simulink model "pendule_inv_capteur_etu"  (R2021a)
settings: Solver=VariableStepAuto  StartTime=0.0  StopTime=100  RelTol=1e-3
values from neighbouring files (symbols this model uses):
  K = [10 1]    [simu_pendule_inv_capteur_etu.m]    (also in simu_pendule_inv_echant_etu.m = [30 10]; simu_pendule_inv_etu.m = [30 10])
  ue = 0    [simu_pendule_inv_capteur_etu.m]    (also in simu_pendule_inv_echant_etu.m; simu_pendule_inv_etu.m)
  x0 = [pi/20 0]'    [simu_pendule_inv_capteur_etu.m]    (also in simu_pendule_inv_echant_etu.m; simu_pendule_inv_etu.m = [pi/10 0]')
  xe = [0 0]'    [simu_pendule_inv_capteur_etu.m]    (also in simu_pendule_inv_echant_etu.m; simu_pendule_inv_etu.m)
settings Model: Creator=ialouane  LastModifiedBy=ialouane

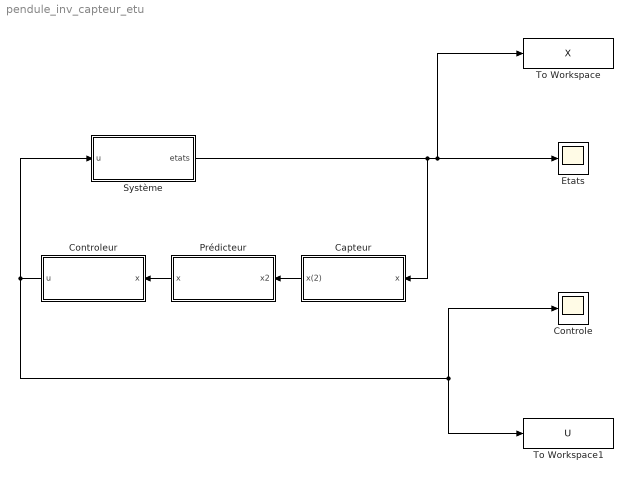
== system pendule_inv_capteur_etu ==
  Capteur : Subsystem
  Controle : Scope
  Controleur : Subsystem
  Etats : Scope
  Prédicteur : Subsystem
  Système : Subsystem
  To Workspace : ToWorkspace  VariableName=X  SaveFormat=Timeseries  SampleTime=-1
  To Workspace1 : ToWorkspace  VariableName=U  SaveFormat=Timeseries  SampleTime=-1
  wires:
  Controleur/1(u) -> Système/1(u), To Workspace1/1, Controle/1
  Système/1(etats) -> Capteur/1(x), To Workspace/1, Etats/1
  Capteur/1(x(2)) -> Prédicteur/1(x2)
  Prédicteur/1(x) -> Controleur/1(x)

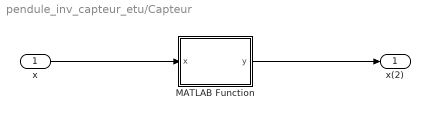
== system pendule_inv_capteur_etu/Capteur ==
  x : Inport
  MATLAB Function : MATLAB Function  TreatAsAtomicUnit=on
  x(2) : Outport
  wires:
  x/1 -> MATLAB Function/1(x)
  MATLAB Function/1(y) -> x(2)/1

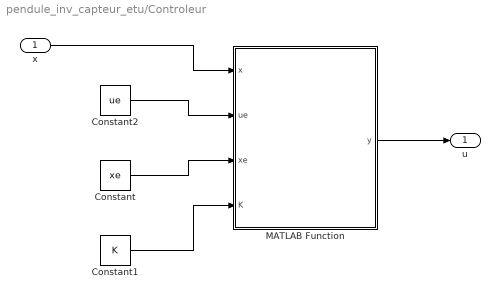
== system pendule_inv_capteur_etu/Controleur ==
  x : Inport
  Constant : Constant  Value=xe
  Constant1 : Constant  Value=K  VectorParams1D=off
  Constant2 : Constant  Value=ue
  MATLAB Function : MATLAB Function  TreatAsAtomicUnit=on
  u : Outport
  wires:
  x/1 -> MATLAB Function/1(x)
  MATLAB Function/1(y) -> u/1
  Constant1/1 -> MATLAB Function/4(K)
  Constant/1 -> MATLAB Function/3(xe)
  Constant2/1 -> MATLAB Function/2(ue)

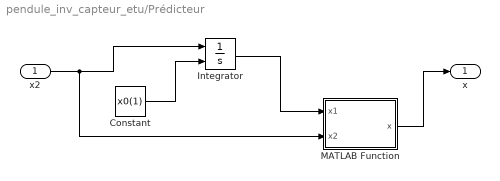
== system pendule_inv_capteur_etu/Prédicteur ==
  x2 : Inport
  Constant : Constant  Value=x0(1)
  Integrator : Integrator  InitialConditionSource=external
  MATLAB Function : MATLAB Function  TreatAsAtomicUnit=on
  x : Outport
  wires:
  Constant/1 -> Integrator/2
  x2/1 -> MATLAB Function/2(x2), Integrator/1
  Integrator/1 -> MATLAB Function/1(x1)
  MATLAB Function/1(x) -> x/1

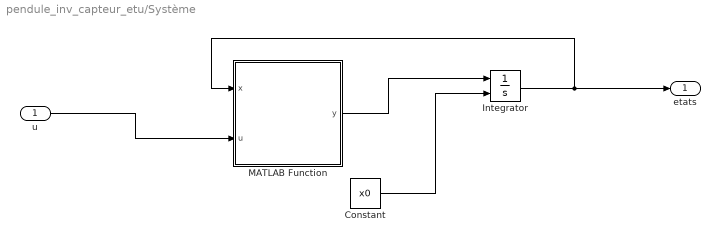
== system pendule_inv_capteur_etu/Système ==
  u : Inport
  Constant : Constant  Value=x0
  Integrator : Integrator  InitialConditionSource=external
  MATLAB Function : MATLAB Function  TreatAsAtomicUnit=on
  etats : Outport
  wires:
  u/1 -> MATLAB Function/2(u)
  MATLAB Function/1(y) -> Integrator/1
  Constant/1 -> Integrator/2
  Integrator/1 -> MATLAB Function/1(x), etats/1

== matlab function pendule_inv_capteur_etu/Controleur/MATLAB Function ==
  data: x input; y output; ue input; xe input; K input
function y = fcn(x,ue,xe,K)
y = ue+(K*(x-xe));

== matlab function pendule_inv_capteur_etu/Système/MATLAB Function ==
  data: x input; u input; y output
function y = fcn(x,u)
l=10;
g=9.81;
y= [x(2);g/l*sin(x(1)) - cos(x(1))*u/l];
end

== matlab function pendule_inv_capteur_etu/Capteur/MATLAB Function ==
  data: x input; y output
function y = fcn(x)
y = x(2);
end

== matlab function pendule_inv_capteur_etu/Prédicteur/MATLAB Function ==
  data: x1 input; x output; x2 input
function x = fcn(x1,x2)
z=zeros(2,1);
z(1)=x1;
z(2)=x2;
x=z;
end
